simulink model "schemat"  (R2022b)
settings: Solver=VariableStepAuto  StartTime=0.0  StopTime=10.0  RelTol=1e-3
values from neighbouring files (symbols this model uses):
  K = [-6.6845,-51.6047,-9.6527,-10]    [main.m]
  Y = [y, 0, 0, 0]'    [main.m]
settings Model: Creator=asialalala  LastModifiedBy=asialalala

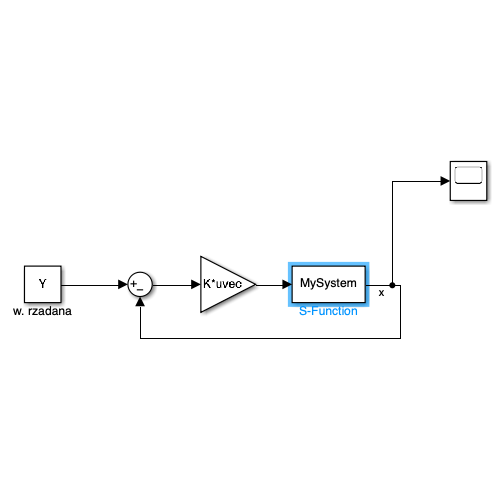
[thumbnail: Simulink's stored preview of the top-level diagram]
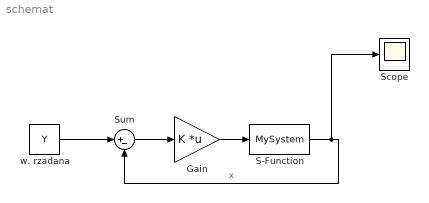
== system schemat ==
  Gain : Gain  Gain=K  Multiplication=Matrix(K*u) (u vector)
  S-Function : S-Function  FunctionName=MySystem  Parameters=state0, params  SFunctionDeploymentMode=off  EnableBusSupport=off
  Scope : Scope
  Sum : Sum  Inputs=|+-
  w. rzadana : Constant  Value=Y
  wires:
  Sum/1 -> Gain/1
  S-Function/1 -> Scope/1, Sum/2  "x"
  w. rzadana/1 -> Sum/1
  Gain/1 -> S-Function/1
